simulink model "model"  (R2020b)
settings: Solver=VariableStepAuto  StartTime=0.0  StopTime=time  MaxStep=1e-3  RelTol=1e-3
values from neighbouring files (symbols this model uses):
  A_plant = [0 1; 880.87 0]    [alternative_model.m]    (also in alternative_model_script.m; observer_convergence.m; p1.m; stable_template.m)
  adj_mtx = [0 0 0 0 0 1 ... (first row only)    [alternative_model.m]    (also in alternative_model_script.m = [0 0 0 0 0 0; epsilon_computation.m = evalin("base", "adj_mtx"); generate_adj_mtx.m = zeros(N); stable_template.m = [0 0 0 0 0 0)
  B_plant = [0; -9.9453]    [alternative_model.m]    (also in alternative_model_script.m; observer_convergence.m; p1.m; stable_template.m)
  C_plant = [708.27 0]    [alternative_model.m]    (also in alternative_model_script.m; observer_convergence.m; p1.m; stable_template.m)
  eps_on = 1    [v1.m]
  K_plant = acker(A_plant, B_plant, poles)    [alternative_model.m]    (also in alternative_model_script.m; p1.m; stable_template.m; template.m)
  output_state = 1    [v1.m]
  png_vct = zeros(N, 1)    [alternative_model.m]    (also in alternative_model_script.m; epsilon_computation.m = evalin("base", "png_vct"); generate_adj_mtx.m = ones(N,1); stable_template.m)
  x0_leader = [1e-3 1e-3]    [alternative_model.m]    (also in alternative_model_script.m; p1.m = [100 0]; stable_template.m = [.1 0]; template.m = [0 0])
  zeta_on = 0    [v1.m]
undefined symbols (not defined in the file or in its folder): epsilon_computation
libraries: dspindex x6, simulink x1
settings Model: Creator=salvo  LastModifiedBy=salvo
settings ModelReferenceCC: ModelReferenceMinAlgLoopOccurrences=on

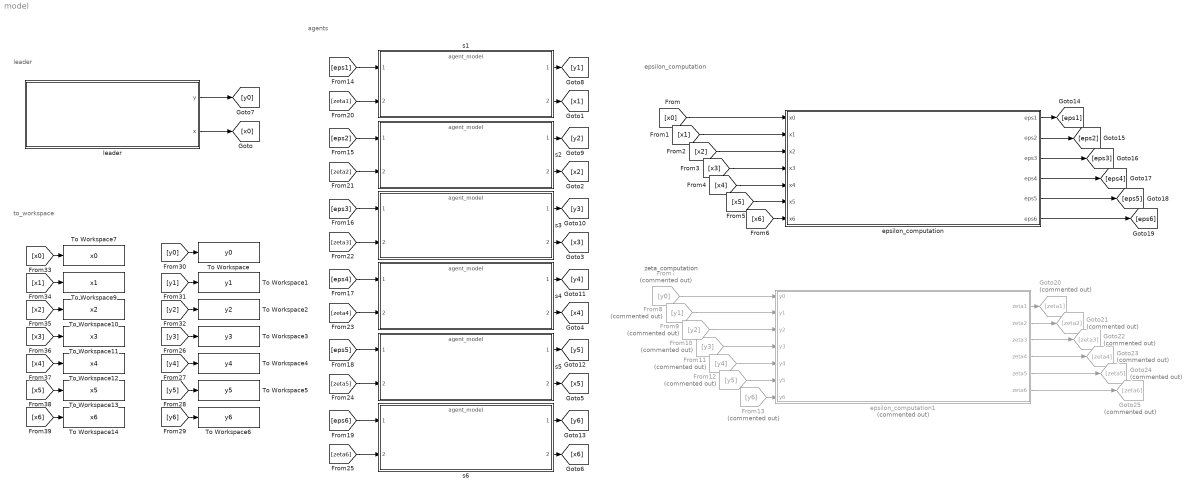
== system model ==
  note: to_workspace
  note: agents
  note: leader
  note: zeta_computation
  note: epsilon_computation
  From10 : From  Commented=on  GotoTag=y3
  From11 : From  Commented=on  GotoTag=y4
  From12 : From  Commented=on  GotoTag=y5
  From13 : From  Commented=on  GotoTag=y6
  From7 : From  Commented=on  GotoTag=y0
  From8 : From  Commented=on  GotoTag=y1
  From9 : From  Commented=on  GotoTag=y2
  Goto20 : Goto  Commented=on  GotoTag=zeta1
  Goto21 : Goto  Commented=on  GotoTag=zeta2
  Goto22 : Goto  Commented=on  GotoTag=zeta3
  Goto23 : Goto  Commented=on  GotoTag=zeta4
  Goto24 : Goto  Commented=on  GotoTag=zeta5
  Goto25 : Goto  Commented=on  GotoTag=zeta6
  To Workspace : ToWorkspace  VariableName=y0  SaveFormat=Timeseries  SampleTime=-1
  To Workspace1 : ToWorkspace  VariableName=y1  SaveFormat=Timeseries  SampleTime=-1
  To Workspace10 : ToWorkspace  VariableName=x2  SaveFormat=Timeseries  SampleTime=-1
  To Workspace11 : ToWorkspace  VariableName=x3  SaveFormat=Timeseries  SampleTime=-1
  To Workspace12 : ToWorkspace  VariableName=x4  SaveFormat=Timeseries  SampleTime=-1
  To Workspace13 : ToWorkspace  VariableName=x5  SaveFormat=Timeseries  SampleTime=-1
  To Workspace14 : ToWorkspace  VariableName=x6  SaveFormat=Timeseries  SampleTime=-1
  To Workspace2 : ToWorkspace  VariableName=y2  SaveFormat=Timeseries  SampleTime=-1
  To Workspace3 : ToWorkspace  VariableName=y3  SaveFormat=Timeseries  SampleTime=-1
  To Workspace4 : ToWorkspace  VariableName=y4  SaveFormat=Timeseries  SampleTime=-1
  To Workspace5 : ToWorkspace  VariableName=y5  SaveFormat=Timeseries  SampleTime=-1
  To Workspace6 : ToWorkspace  VariableName=y6  SaveFormat=Timeseries  SampleTime=-1
  To Workspace7 : ToWorkspace  VariableName=x0  SaveFormat=Timeseries  SampleTime=-1
  To Workspace9 : ToWorkspace  VariableName=x1  SaveFormat=Timeseries  SampleTime=-1
  epsilon_computation : Subsystem
  epsilon_computation1 : Subsystem  Commented=on
  leader : Subsystem
  s{1..6} (6 alike) : ModelReference  ModelNameDialog=agent_model  SimulationMode=Normal  ModelReferenceVersion=1.21
  wires:
  leader/2(x) -> [x0]
  s1/2 -> [x1]
  s2/2 -> [x2]
  s3/2 -> [x3]
  s4/2 -> [x4]
  s5/2 -> [x5]
  s6/2 -> [x6]
  [x0] -> epsilon_computation/1(x0)
  [x1] -> epsilon_computation/2(x1)
  [x3] -> epsilon_computation/4(x3)
  [x2] -> epsilon_computation/3(x2)
  [x4] -> epsilon_computation/5(x4)
  [x5] -> epsilon_computation/6(x5)
  [x6] -> epsilon_computation/7(x6)
  leader/1(y) -> [y0]
  s1/1 -> [y1]
  s2/1 -> [y2]
  s3/1 -> [y3]
  s4/1 -> [y4]
  s5/1 -> [y5]
  s6/1 -> [y6]
  From9/1 -> epsilon_computation1/3(y2)
  From7/1 -> epsilon_computation1/1(y0)
  From8/1 -> epsilon_computation1/2(y1)
  From11/1 -> epsilon_computation1/5(y4)
  From10/1 -> epsilon_computation1/4(y3)
  From13/1 -> epsilon_computation1/7(y6)
  From12/1 -> epsilon_computation1/6(y5)
  epsilon_computation/1(eps1) -> [eps1]
  epsilon_computation/2(eps2) -> [eps2]
  epsilon_computation/3(eps3) -> [eps3]
  epsilon_computation/4(eps4) -> [eps4]
  epsilon_computation/5(eps5) -> [eps5]
  epsilon_computation/6(eps6) -> [eps6]
  epsilon_computation1/4(zeta4) -> Goto23/1
  epsilon_computation1/3(zeta3) -> Goto22/1
  epsilon_computation1/6(zeta6) -> Goto25/1
  epsilon_computation1/2(zeta2) -> Goto21/1
  epsilon_computation1/5(zeta5) -> Goto24/1
  epsilon_computation1/1(zeta1) -> Goto20/1
  [eps1] -> s1/1
  [eps4] -> s4/1
  [eps3] -> s3/1
  [eps2] -> s2/1
  [eps5] -> s5/1
  [eps6] -> s6/1
  [zeta1] -> s1/2
  [zeta2] -> s2/2
  [zeta3] -> s3/2
  [zeta4] -> s4/2
  [zeta5] -> s5/2
  [zeta6] -> s6/2
  [y6] -> To Workspace6/1
  [y5] -> To Workspace5/1
  [y0] -> To Workspace/1
  [y1] -> To Workspace1/1
  [y2] -> To Workspace2/1
  [y3] -> To Workspace3/1
  [y4] -> To Workspace4/1
  [x6] -> To Workspace14/1
  [x5] -> To Workspace13/1
  [x4] -> To Workspace12/1
  [x3] -> To Workspace11/1
  [x1] -> To Workspace9/1
  [x2] -> To Workspace10/1
  [x0] -> To Workspace7/1

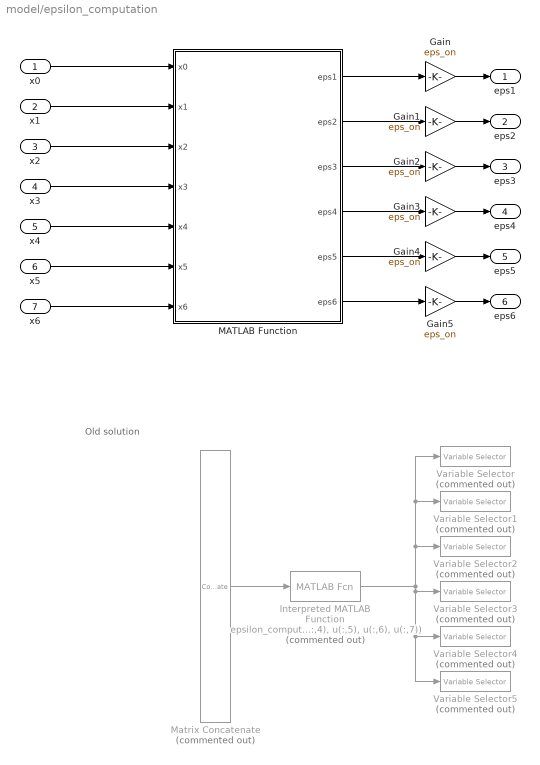
== system model/epsilon_computation ==
  note: Old solution
  x0 : Inport  PortDimensions=[2,1]
  x1 : Inport  Port=2  PortDimensions=[2,1]
  x2 : Inport  Port=3  PortDimensions=[2,1]
  x3 : Inport  Port=4  PortDimensions=[2,1]
  x4 : Inport  Port=5  PortDimensions=[2,1]
  x5 : Inport  Port=6  PortDimensions=[2,1]
  x6 : Inport  Port=7  PortDimensions=[2,1]
  Gain{,1..5} (6 alike) : Gain  Gain=eps_on
  Interpreted MATLAB Function : MATLABFcn  Commented=on  MATLABFcn=epsilon_computation(u(:,1), u(:,2), u(:,3), u(:,4), u(:,5), u(:,6), u(:,7))  Output1D=off
  MATLAB Function : MATLAB Function  TreatAsAtomicUnit=on
  Matrix Concatenate : Concatenate  Commented=on  NumInputs=7  Mode=Multidimensional array  ConcatenateDimension=2
  Variable Selector : dspindex/Variable Selector  Commented=on  NumInputs=1  rowsOrCols=Columns  IdxMode=Fixed  Elements=1  ZerOneIdxMode=One-based  errmode=Clip Index  FillMode=on  FillValues=0
  Variable Selector1 : dspindex/Variable Selector  Commented=on  NumInputs=1  rowsOrCols=Columns  IdxMode=Fixed  Elements=2  ZerOneIdxMode=One-based  errmode=Clip Index  FillMode=on  FillValues=0
  Variable Selector2 : dspindex/Variable Selector  Commented=on  NumInputs=1  rowsOrCols=Columns  IdxMode=Fixed  Elements=3  ZerOneIdxMode=One-based  errmode=Clip Index  FillMode=on  FillValues=0
  Variable Selector3 : dspindex/Variable Selector  Commented=on  NumInputs=1  rowsOrCols=Columns  IdxMode=Fixed  Elements=4  ZerOneIdxMode=One-based  errmode=Clip Index  FillMode=on  FillValues=0
  Variable Selector4 : dspindex/Variable Selector  Commented=on  NumInputs=1  rowsOrCols=Columns  IdxMode=Fixed  Elements=5  ZerOneIdxMode=One-based  errmode=Clip Index  FillMode=on  FillValues=0
  Variable Selector5 : dspindex/Variable Selector  Commented=on  NumInputs=1  rowsOrCols=Columns  IdxMode=Fixed  Elements=6  ZerOneIdxMode=One-based  errmode=Clip Index  FillMode=on  FillValues=0
  eps1 : Outport
  eps2 : Outport  Port=2
  eps3 : Outport  Port=3
  eps4 : Outport  Port=4
  eps5 : Outport  Port=5
  eps6 : Outport  Port=6
  wires:
  Gain/1 -> eps1/1
  Gain1/1 -> eps2/1
  Gain2/1 -> eps3/1
  Gain3/1 -> eps4/1
  Gain4/1 -> eps5/1
  Gain5/1 -> eps6/1
  Matrix Concatenate/1 -> Interpreted MATLAB Function/1
  Interpreted MATLAB Function/1 -> Variable Selector5/1, Variable Selector4/1, Variable Selector3/1, Variable Selector2/1, Variable Selector1/1, Variable Selector/1
  x0/1 -> MATLAB Function/1(x0)
  x1/1 -> MATLAB Function/2(x1)
  x2/1 -> MATLAB Function/3(x2)
  x3/1 -> MATLAB Function/4(x3)
  x4/1 -> MATLAB Function/5(x4)
  x5/1 -> MATLAB Function/6(x5)
  x6/1 -> MATLAB Function/7(x6)
  MATLAB Function/1(eps1) -> Gain/1
  MATLAB Function/2(eps2) -> Gain1/1
  MATLAB Function/3(eps3) -> Gain2/1
  MATLAB Function/4(eps4) -> Gain3/1
  MATLAB Function/5(eps5) -> Gain4/1
  MATLAB Function/6(eps6) -> Gain5/1

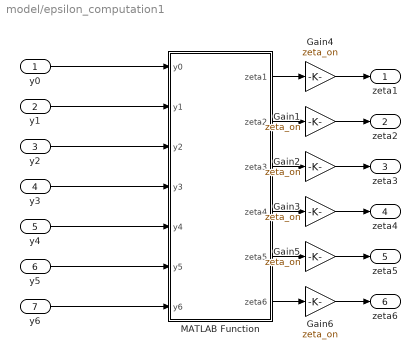
== system model/epsilon_computation1 ==
  y0 : Inport
  y1 : Inport  Port=2
  y2 : Inport  Port=3
  y3 : Inport  Port=4
  y4 : Inport  Port=5
  y5 : Inport  Port=6
  y6 : Inport  Port=7
  Gain{1..6} (6 alike) : Gain  Gain=zeta_on
  MATLAB Function : MATLAB Function  TreatAsAtomicUnit=on
  zeta1 : Outport
  zeta2 : Outport  Port=2
  zeta3 : Outport  Port=3
  zeta4 : Outport  Port=4
  zeta5 : Outport  Port=5
  zeta6 : Outport  Port=6
  wires:
  y0/1 -> MATLAB Function/1(y0)
  y1/1 -> MATLAB Function/2(y1)
  y2/1 -> MATLAB Function/3(y2)
  y3/1 -> MATLAB Function/4(y3)
  y4/1 -> MATLAB Function/5(y4)
  y5/1 -> MATLAB Function/6(y5)
  y6/1 -> MATLAB Function/7(y6)
  MATLAB Function/2(zeta2) -> Gain1/1
  MATLAB Function/1(zeta1) -> Gain4/1
  MATLAB Function/3(zeta3) -> Gain2/1
  MATLAB Function/4(zeta4) -> Gain3/1
  MATLAB Function/5(zeta5) -> Gain5/1
  MATLAB Function/6(zeta6) -> Gain6/1
  Gain4/1 -> zeta1/1
  Gain1/1 -> zeta2/1
  Gain2/1 -> zeta3/1
  Gain3/1 -> zeta4/1
  Gain5/1 -> zeta5/1
  Gain6/1 -> zeta6/1

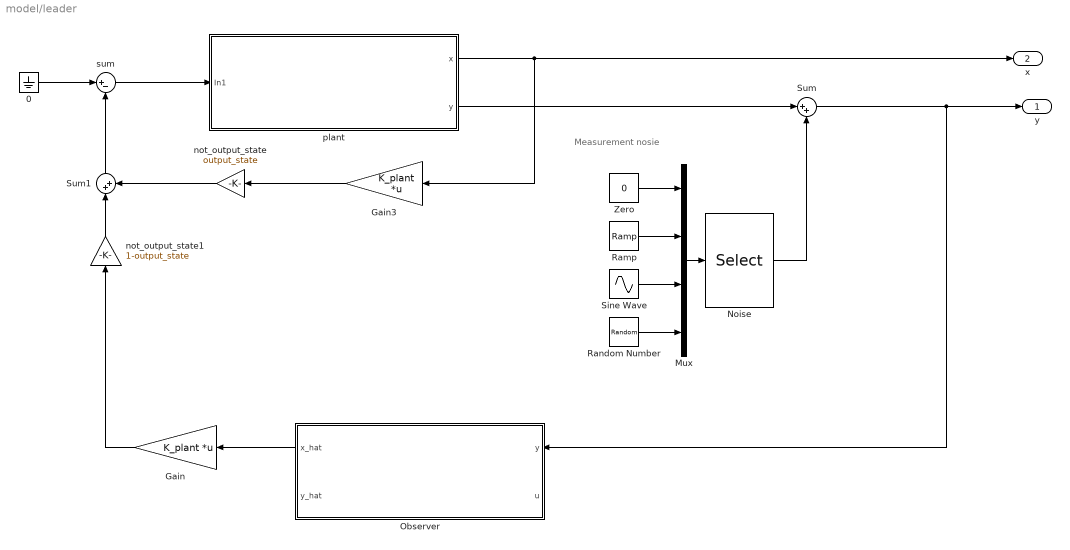
== system model/leader ==
  note: Measurement nosie
  0 : Ground
  Gain : Gain  Gain=K_plant  Multiplication=Matrix(K*u)
  Gain3 : Gain  Gain=K_plant  Multiplication=Matrix(K*u)
  Mux : Mux
  Noise : Selector  InputPortWidth=4  IndexOptions=Index vector (dialog)  Indices=measurement_noise_type  OutputSizes=1
  Observer : Subsystem
  Ramp : simulink/Sources/Ramp  slope=1  start=0  InitialOutput=0
  Random Number : RandomNumber  SampleTime=0.1
  Sine Wave : Sin  SampleTime=0
  Sum : Sum  Inputs=|++
  Sum1 : Sum  Inputs=|++
  Zero : Constant  Value=0  OutDataTypeStr=Inherit: Inherit via back propagation
  not_output_state : Gain  Gain=output_state
  not_output_state1 : Gain  Gain=1-output_state
  plant : Subsystem
  sum : Sum  Inputs=|+-
  y : Outport
  x : Outport  Port=2
  wires:
  plant/2(y) -> Sum/1
  sum/1 -> plant/1(In1)
  Observer/1(x_hat) -> Gain/1
  0/1 -> sum/1
  Sum1/1 -> sum/2
  Gain3/1 -> not_output_state/1
  Gain/1 -> not_output_state1/1
  plant/1(x) -> x/1, Gain3/1
  not_output_state/1 -> Sum1/2
  not_output_state1/1 -> Sum1/1
  Sum/1 -> Observer/1(y), y/1
  Noise/1 -> Sum/2
  Mux/1 -> Noise/1
  Ramp/1 -> Mux/2
  Sine Wave/1 -> Mux/3
  Random Number/1 -> Mux/4
  Zero/1 -> Mux/1

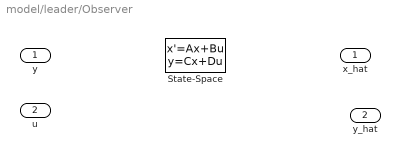
== system model/leader/Observer ==
  y : Inport
  u : Inport  Port=2
  State-Space : StateSpace  InitialCondition=0
  x_hat : Outport
  y_hat : Outport  Port=2

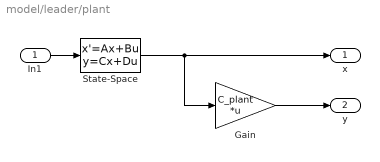
== system model/leader/plant ==
  In1 : Inport
  Gain : Gain  Gain=C_plant  Multiplication=Matrix(K*u)
  State-Space : StateSpace  A=A_plant  B=B_plant  C=eye(2)  D=[0; 0]  InitialCondition=x0_leader
  x : Outport  PortDimensions=[2,1]
  y : Outport  Port=2  PortDimensions=1
  wires:
  In1/1 -> State-Space/1
  Gain/1 -> y/1
  State-Space/1 -> x/1, Gain/1

== matlab function model/epsilon_computation1/MATLAB Function ==
  data: y0 input; zeta1 output; y1 input; y2 input; y3 input; y4 input; y5 input; y6 input; zeta2 output; zeta3 output; zeta4 output; zeta5 output; zeta6 output
function [zeta1, zeta2, zeta3, zeta4, zeta5, zeta6] = fcn(y0, y1, y2, y3, y4, y5, y6)

N = 6;
for i =  1:N
    e = 0; % zeta
    e = e + png_vct(i) * (y0 - eval('y'+i)); % pinning gain
    for j = 1:N
       e = e + adj_mtx(i,j) * ( eval('y'+j) - eval('y'+i) ); % edge gain
    end
    eval('zeta'+i+'=e');
end

== matlab function model/epsilon_computation/MATLAB Function ==
  data: x0 input; eps1 output; x1 input; x2 input; x3 input; x4 input; x5 input; x6 input; png_vct parameter; adj_mtx parameter; eps2 output; eps3 output; eps4 output; eps5 output; eps6 output
function [eps1, eps2, eps3, eps4, eps5, eps6] = epsilon_computation(x0, x1, x2, x3, x4, x5, x6, png_vct, adj_mtx)

N = 6;

eps = zeros(N, 2);
x = [x1 x2 x3 x4 x5 x6];
for i = 1:N
    e = [0; 0]; %epsilon
    e = e + png_vct(i) .* (x0 - x(:,i)); % pinning gain
    for j = 1:N
       e = e + adj_mtx(i,j) .* ( x(:,j) - x(:,i) ); % edge gain
    end
    eps(i,:) = e;
end

eps1 = eps(1,:);
eps2 = eps(2,:);
eps3 = eps(3,:);
eps4 = eps(4,:);
eps5 = eps(5,:);
eps6 = eps(6,:);

end
